simulink model "invertedpd"  (Simulink 5.0)
settings: Solver=ode1  SolverMode=SingleTasking  StartTime=0.0  StopTime=70.0  FixedStep=0.001  RelTol=1e-3
libraries: pci1711 x3
settings Model: LastModifiedBy=AD  ExtModeMexFile=rtwinext  ExtModeTrigMode=oneshot  ExtModeTrigDuration=100000  ExtModeLogAll=off  SimulationMode=external  LimitDataPoints=off  BlockReductionOpt=off  BooleanDataType=off  RTWSystemTargetFile=rtwinfbk.tlc  RTWTemplateMakefile=winfbktmf  RTWOptions="-aCCOptimize=1 -aEnforceIntegerDowncast=1 -aExtMode=1 -aFoldNonRolledExpr=1 -aForceParamTrailComments=0 -aGenerateComments=1 -aGenerateReport=0 -aIncDataTypeInIds=0 -aIncHierarchyInIds=0 -aInlineInvariantSignals=0 -aInlineParameters=0 -aInlinedPrmAccess=\"Literals\" -aLocalBlockOutputs=1 -aMaxRTWIdLen=31 -aPrefixModelToSubsysFcnNames=1 -aRTWVerbose=1 -aRebuildAll=0 -aRollThreshold=5 -aShowEliminatedStatements=1"

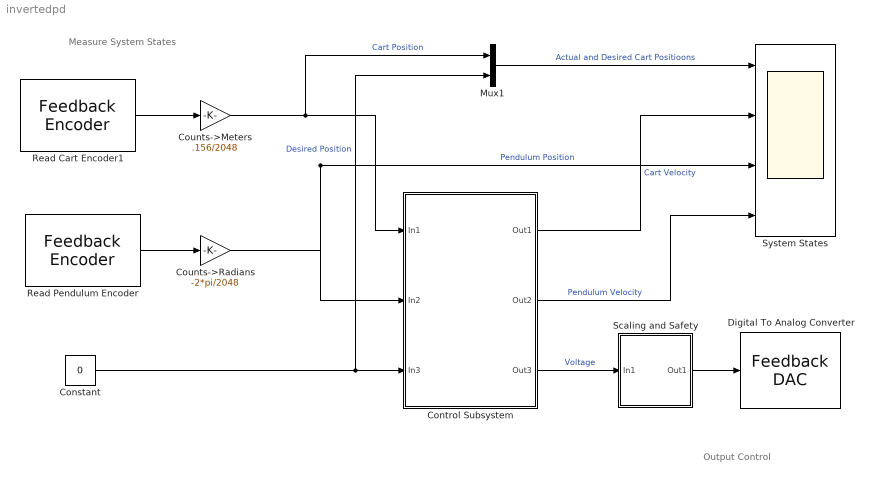
== system invertedpd ==
  note: Measure System States
  note: Output Control
  Constant : Constant  Value=0
  Control Subsystem : Subsystem
  Counts->Meters : Gain  Gain=.156/2048  SaturateOnIntegerOverflow=on
  Counts->Radians : Gain  Gain=-2*pi/2048  SaturateOnIntegerOverflow=on
  Digital To Analog Converter : pci1711/Advantech  PCI1711 I//O Board Lib/Feedback DAC  channel=0  range=0  tsamp=0.001  hwAccess=on
  Mux1 : Mux  Inputs=2
  Read Cart Encoder1 : pci1711/Advantech  PCI1711 I//O Board Lib/Feedback Encoder   channel=0  offset=0  tsamp=0.001  hwAccess=on
  Read Pendulum Encoder : pci1711/Advantech  PCI1711 I//O Board Lib/Feedback Encoder   channel=1  offset=-1024  tsamp=0.001  hwAccess=on
  Scaling and Safety : Subsystem
  System States : Scope  NumInputPorts=4
      settings: TimeRange=70  YMin=-0.5~-1~-6~-15  YMax=0.5~1~6~15  Decimation=0.1  SampleInput=on  SampleTime=0.01
  wires:
  Counts->Meters/1 -> Mux1/1, Control Subsystem/1(In1)  "Cart Position"
  Counts->Radians/1 -> System States/3, Control Subsystem/2(In2)  "Pendulum Position"
  Scaling and Safety/1(Out1) -> Digital To Analog Converter/1
  Constant/1 -> Mux1/2, Control Subsystem/3(In3)  "Desired Position"
  Control Subsystem/3(Out3) -> Scaling and Safety/1(In1)  "Voltage"
  Mux1/1 -> System States/1  "Actual and Desired Cart Positioons"
  Read Cart Encoder1/1 -> Counts->Meters/1
  Read Pendulum Encoder/1 -> Counts->Radians/1
  Control Subsystem/1(Out1) -> System States/2  "Cart Velocity"
  Control Subsystem/2(Out2) -> System States/4  "Pendulum Velocity"

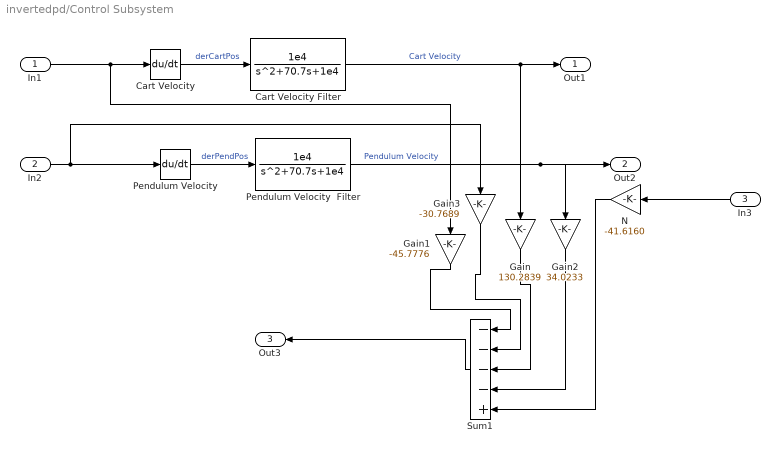
== system invertedpd/Control Subsystem ==
  In1 : Inport
  In2 : Inport  Port=2
  In3 : Inport  Orientation=left  Port=3
  Cart Velocity : Derivative
  Cart Velocity Filter : TransferFcn  Numerator=[1e4]  Denominator=[1 70.7 1e4]
  Gain : Gain  Orientation=down  Gain=130.2839  SaturateOnIntegerOverflow=on
  Gain1 : Gain  Orientation=down  Gain=-45.7776  SaturateOnIntegerOverflow=on
  Gain2 : Gain  Orientation=down  Gain=34.0233  SaturateOnIntegerOverflow=on
  Gain3 : Gain  Orientation=down  Gain=-30.7689  SaturateOnIntegerOverflow=on
  N : Gain  Orientation=left  Gain=-41.6160  SaturateOnIntegerOverflow=on
  Pendulum Velocity : Derivative
  Pendulum Velocity  Filter : TransferFcn  Numerator=[1e4]  Denominator=[1 70.7 1e4]
  Sum1 : Sum  Orientation=left  Inputs=----+  SaturateOnIntegerOverflow=on  InputSameDT=on
  Out1 : Outport
  Out2 : Outport  Port=2
  Out3 : Outport  Orientation=left  Port=3
  wires:
  Cart Velocity/1 -> Cart Velocity Filter/1  "derCartPos"
  Pendulum Velocity/1 -> Pendulum Velocity  Filter/1  "derPendPos"
  Cart Velocity Filter/1 -> Out1/1, Gain/1  "Cart Velocity"
  Pendulum Velocity  Filter/1 -> Out2/1, Gain2/1  "Pendulum Velocity"
  In1/1 -> Cart Velocity/1, Gain1/1
  In2/1 -> Pendulum Velocity/1, Gain3/1
  Gain1/1 -> Sum1/1
  Gain/1 -> Sum1/3
  Gain3/1 -> Sum1/2
  Gain2/1 -> Sum1/4
  Sum1/1 -> Out3/1
  N/1 -> Sum1/5
  In3/1 -> N/1

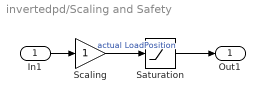
== system invertedpd/Scaling and Safety ==
  In1 : Inport
  Saturation : Saturate  UpperLimit=2.5  LowerLimit=-2.5
  Scaling : Gain  SaturateOnIntegerOverflow=on
  Out1 : Outport
  wires:
  Saturation/1 -> Out1/1
  In1/1 -> Scaling/1
  Scaling/1 -> Saturation/1  "actual LoadPosition"
